simulink model "TPCH1"  (Simulink 5.0)
settings: Solver=ode45  StartTime=0.0  StopTime=0.35  RelTol=1e-3
libraries: powerlib_extras x1
settings Model: LastModifiedBy=Blue Phoenix  BlockReductionOpt=off  BooleanDataType=off

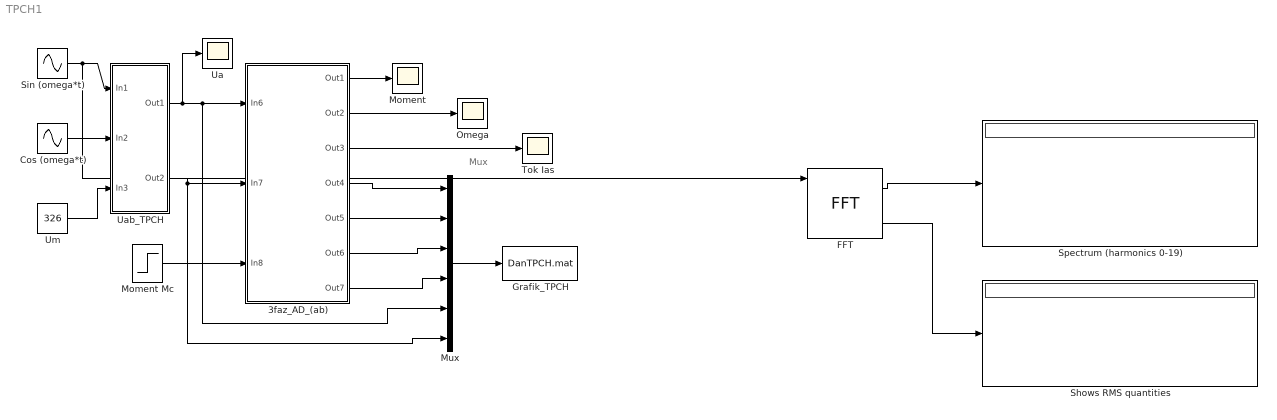
== system TPCH1 ==
  note: Mux
  " 3faz_AD_(ab)" : Subsystem
  Cos (omega*t) : Sin  Frequency=314*0.5  Phase=-pi/2  SampleTime=0
  FFT : powerlib_extras/Discrete Measurements/FFT  f1=50  Ts=500e-6  TsFFT=0.1  base="[1 1  1]"  nDec=0  mask=[1 -1 1]  figure_N=1
  Grafik_TPCH : ToFile  Filename=DanTPCH.mat
  Moment : Scope
      settings: TickLabels=on  TimeRange=80  YMin=-1  YMax=2  DataFormat=Array
  Moment Mc : Step  Time=0.06  Before=0.0  After=17  SampleTime=0
  Mux : Mux  Inputs=6
  Omega : Scope
      settings: TickLabels=on  TimeRange=0.2  YMin=-50  YMax=350  DataFormat=Array
  Shows RMS quantities : Display
      settings: Format=bank
  Sin (omega*t) : Sin  Frequency=314*0.5  SampleTime=0
  Spectrum (harmonics 0-19) : Display
      settings: Format=bank
  Tok Ias : Scope
      settings: TickLabels=on  TimeRange=80  YMin=-1  YMax=2  SaveName=ScopeData2  DataFormat=Array
  Ua : Scope
      settings: TickLabels=on  TimeRange=80  YMin=-1  YMax=2  SaveName=ScopeData3  DataFormat=Array
  Uab_TPCH : Subsystem
  Um : Constant  Value=326
  wires:
  " 3faz_AD_(ab)"/1(Out1) -> Moment/1
  " 3faz_AD_(ab)"/2(Out2) -> Omega/1
  " 3faz_AD_(ab)"/3(Out3) -> Tok Ias/1
  Uab_TPCH/1(Out1) -> " 3faz_AD_(ab)"/1(In6), Mux/5, Ua/1
  Uab_TPCH/2(Out2) -> Mux/6, " 3faz_AD_(ab)"/2(In7)
  " 3faz_AD_(ab)"/4(Out4) -> Mux/1
  " 3faz_AD_(ab)"/5(Out5) -> Mux/2
  " 3faz_AD_(ab)"/6(Out6) -> Mux/3
  " 3faz_AD_(ab)"/7(Out7) -> Mux/4
  Mux/1 -> Grafik_TPCH/1
  Moment Mc/1 -> " 3faz_AD_(ab)"/3(In8)
  Sin (omega*t)/1 -> Uab_TPCH/1(In1), FFT/1
  Cos (omega*t)/1 -> Uab_TPCH/2(In2)
  Um/1 -> Uab_TPCH/3(In3)
  FFT/2 -> Shows RMS quantities/1
  FFT/1 -> Spectrum (harmonics 0-19)/1

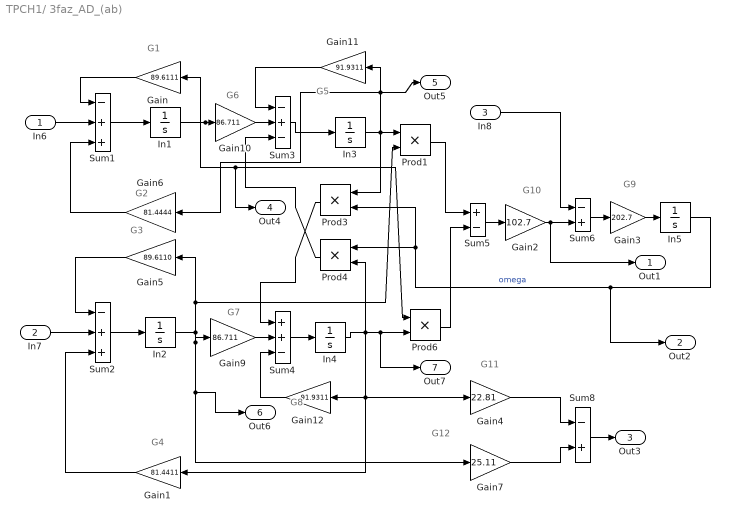
== system TPCH1/ 3faz_AD_(ab) ==
  note: G1
  note: G2
  note: G3
  note: G4
  note: G10
  note: G9
  note: G6
  note: G7
  note: G8
  note: G5
  note: G11
  note: G12
  In6 : Inport
  In7 : Inport  Port=2
  In8 : Inport  Port=3
  "  Prod1" : Product  SaturateOnIntegerOverflow=on  InputSameDT=on
  Gain : Gain  Orientation=left  Gain=89.6111  SaturateOnIntegerOverflow=on
  Gain1 : Gain  Orientation=left  Gain=81.4411  SaturateOnIntegerOverflow=on
  Gain10 : Gain  Gain=86.711  SaturateOnIntegerOverflow=on
  Gain11 : Gain  Orientation=left  Gain=91.9311  SaturateOnIntegerOverflow=on
  Gain12 : Gain  Orientation=left  Gain=91.9311  SaturateOnIntegerOverflow=on
  Gain2 : Gain  Gain=102.7  SaturateOnIntegerOverflow=on
  Gain3 : Gain  Gain=202.7  SaturateOnIntegerOverflow=on
  Gain4 : Gain  Gain=22.81  SaturateOnIntegerOverflow=on
  Gain5 : Gain  Orientation=left  Gain=89.6110  SaturateOnIntegerOverflow=on
  Gain6 : Gain  Orientation=left  Gain=81.4444  SaturateOnIntegerOverflow=on
  Gain7 : Gain  Gain=25.11  SaturateOnIntegerOverflow=on
  Gain9 : Gain  Gain=86.711  SaturateOnIntegerOverflow=on
  In{1..5} (5 alike) : Integrator
  Prod3 : Product  Orientation=left  SaturateOnIntegerOverflow=on  InputSameDT=on
  Prod4 : Product  Orientation=left  SaturateOnIntegerOverflow=on  InputSameDT=on
  Prod6 : Product  SaturateOnIntegerOverflow=on  InputSameDT=on
  Sum1 : Sum  Inputs=-++  SaturateOnIntegerOverflow=on  InputSameDT=on
  Sum2 : Sum  Inputs=-++  SaturateOnIntegerOverflow=on  InputSameDT=on
  Sum3 : Sum  Inputs=-+-  SaturateOnIntegerOverflow=on  InputSameDT=on
  Sum4 : Sum  Inputs=++-  SaturateOnIntegerOverflow=on  InputSameDT=on
  Sum5 : Sum  Inputs=+-  SaturateOnIntegerOverflow=on  InputSameDT=on
  Sum6 : Sum  Inputs=-+  SaturateOnIntegerOverflow=on  InputSameDT=on
  Sum8 : Sum  Inputs=-+  SaturateOnIntegerOverflow=on  InputSameDT=on
  Out1 : Outport
  Out2 : Outport  Port=2
  Out3 : Outport  Port=3
  Out4 : Outport  Port=4
  Out5 : Outport  Port=5
  Out6 : Outport  Port=6
  Out7 : Outport  Port=7
  wires:
  Gain/1 -> Sum1/1
  Sum2/1 -> In2/1
  In4/1 -> Prod4/2, Gain1/1, Gain12/1, Gain4/1, Prod6/2, Out7/1
  In3/1 -> Prod3/1, "  Prod1"/1, Gain6/1, Gain11/1, Out5/1
  Prod6/1 -> Sum5/2
  Gain3/1 -> In5/1
  In8/1 -> Sum6/1
  "  Prod1"/1 -> Sum5/1
  Sum3/1 -> In3/1
  Sum5/1 -> Gain2/1
  Sum1/1 -> In1/1
  In2/1 -> "  Prod1"/2, Gain5/1, Gain9/1, Gain7/1, Out6/1
  In1/1 -> Gain10/1, Gain/1, Prod6/1, Out4/1
  Gain10/1 -> Sum3/2
  Gain9/1 -> Sum4/2
  Gain5/1 -> Sum2/1
  Prod4/1 -> Sum3/3
  Prod3/1 -> Sum4/1
  Gain2/1 -> Sum6/2, Out1/1
  Gain11/1 -> Sum3/1
  Gain12/1 -> Sum4/3
  In5/1 -> Prod3/2, Prod4/1, Out2/1  "omega"
  Sum4/1 -> In4/1
  Gain7/1 -> Sum8/2
  Gain4/1 -> Sum8/1
  Gain6/1 -> Sum1/3
  Gain1/1 -> Sum2/3
  In7/1 -> Sum2/2
  In6/1 -> Sum1/2
  Sum8/1 -> Out3/1
  Sum6/1 -> Gain3/1

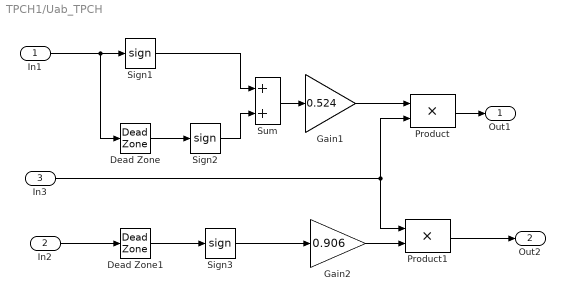
== system TPCH1/Uab_TPCH ==
  In1 : Inport
  In2 : Inport  Port=2
  In3 : Inport  Port=3
  Dead Zone : DeadZone  LowerValue=-0.866  UpperValue=0.866  SaturateOnIntegerOverflow=on
  Dead Zone1 : DeadZone  SaturateOnIntegerOverflow=on
  Gain1 : Gain  Gain=0.524  SaturateOnIntegerOverflow=on
  Gain2 : Gain  Gain=0.906  SaturateOnIntegerOverflow=on
  Product : Product  SaturateOnIntegerOverflow=on  InputSameDT=on
  Product1 : Product  SaturateOnIntegerOverflow=on  InputSameDT=on
  Sign1 : Signum
  Sign2 : Signum
  Sign3 : Signum
  Sum : Sum  SaturateOnIntegerOverflow=on  InputSameDT=on
  Out1 : Outport
  Out2 : Outport  Port=2
  wires:
  In1/1 -> Sign1/1, Dead Zone/1
  Sign1/1 -> Sum/1
  Dead Zone/1 -> Sign2/1
  Sign2/1 -> Sum/2
  In2/1 -> Dead Zone1/1
  Dead Zone1/1 -> Sign3/1
  Sum/1 -> Gain1/1
  Sign3/1 -> Gain2/1
  Gain1/1 -> Product/1
  Product/1 -> Out1/1
  Gain2/1 -> Product1/2
  Product1/1 -> Out2/1
  In3/1 -> Product/2, Product1/1
